simulink library "libreria_comunicaciones_cliente1T"  (R2018a)
settings: Solver=VariableStepAuto  StartTime=0.0  StopTime=10.0  RelTol=1e-3
undefined symbols (not defined in the file or in its folder): Ts
libraries: simulink x1
settings Model: Creator=ana-n  LastModifiedBy=ana-n
settings CodeAppCC: StateflowObjectComments=on

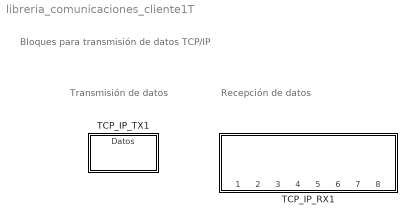
== system libreria_comunicaciones_cliente1T ==
  note: Bloques para transmisión de datos TCP/IP
  note: Recepción de datos
  note: Transmisión de datos
  TCP_IP_RX1 : Subsystem
      mask Display:
      | disp('TCP_IP_RX')
      | port_label('output',1,'RL1');
      | port_label('output',2,'RL2');
      | port_label('output',3,'RL3');
      | port_label('output',4,'RL4');
      | port_label('output',5,'RL5');
      | port_label('output',6,'Top');
      | port_label('output',7,'Top_graf');
      | port_label('output',8,'add');
  TCP_IP_TX1 : Subsystem
      mask Display: disp('TCP_IP_TX');

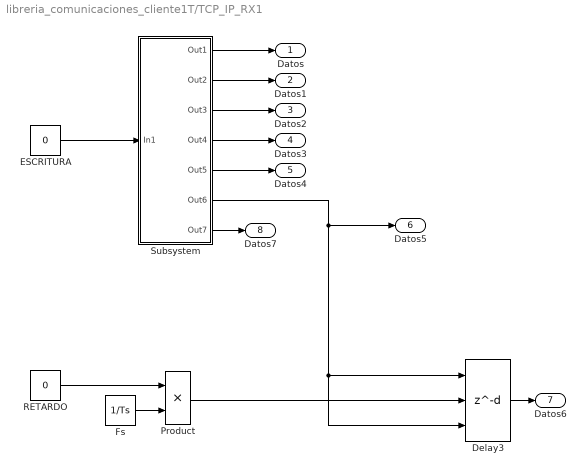
== system libreria_comunicaciones_cliente1T/TCP_IP_RX1 ==
  Delay3 : Delay  DelayLengthSource=Input port  DelayLength=1  DelayLengthUpperLimit=1000  InitialConditionSource=Input port  InitialCondition=0  InputProcessing=Inherited
      settings: InputPortMap=u0,p1,p4
  ESCRITURA : Constant  Value=0
  Fs : Constant  Value=1/Ts
  Product : Product
  RETARDO : Constant  Value=0
  Subsystem : Subsystem
      mask Display: disp('demux')
  Datos : Outport
  Datos1 : Outport  Port=2
  Datos2 : Outport  Port=3
  Datos3 : Outport  Port=4
  Datos4 : Outport  Port=5
  Datos5 : Outport  Port=6
  Datos6 : Outport  Port=7
  Datos7 : Outport  Port=8
  wires:
  Product/1 -> Delay3/2
  RETARDO/1 -> Product/1
  Fs/1 -> Product/2
  ESCRITURA/1 -> Subsystem/1(In1)
  Subsystem/1(Out1) -> Datos/1
  Subsystem/2(Out2) -> Datos1/1
  Subsystem/3(Out3) -> Datos2/1
  Subsystem/4(Out4) -> Datos3/1
  Subsystem/5(Out5) -> Datos4/1
  Subsystem/6(Out6) -> Datos5/1, Delay3/1, Delay3/3
  Delay3/1 -> Datos6/1
  Subsystem/7(Out7) -> Datos7/1

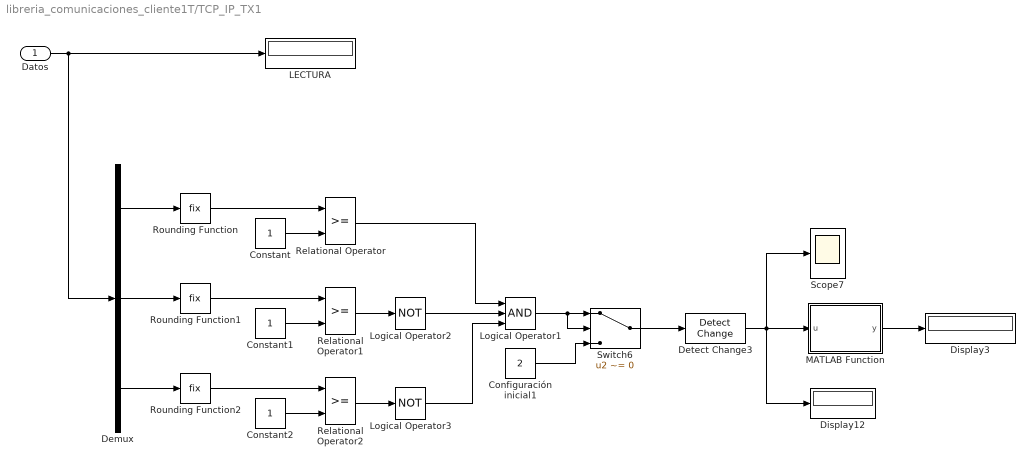
== system libreria_comunicaciones_cliente1T/TCP_IP_TX1 ==
  Datos : Inport
  Configuración inicial1 : Constant  Value=2
  Constant : Constant
  Constant1 : Constant
  Constant2 : Constant
  Demux : Demux  Outputs=3
  Detect Change3 : simulink/Logic and Bit Operations/Detect Change  vinit=0  OutDataTypeStr=boolean
  Display12 : Display
  Display3 : Display
  LECTURA : Display
  Logical Operator1 : Logic  Inputs=3  AllPortsSameDT=off  OutDataTypeStr=boolean
  Logical Operator2 : Logic  Operator=NOT  Inputs=3  AllPortsSameDT=off  OutDataTypeStr=boolean
  Logical Operator3 : Logic  Operator=NOT  Inputs=3  AllPortsSameDT=off  OutDataTypeStr=boolean
  MATLAB Function : MATLAB Function  TreatAsAtomicUnit=on
  Relational Operator : RelationalOperator  OutDataTypeStr=boolean  RndMeth=Simplest
  Relational Operator1 : RelationalOperator  OutDataTypeStr=boolean  RndMeth=Simplest
  Relational Operator2 : RelationalOperator  OutDataTypeStr=boolean  RndMeth=Simplest
  Rounding Function : Rounding  Operator=fix
  Rounding Function1 : Rounding  Operator=fix
  Rounding Function2 : Rounding  Operator=fix
  Scope7 : Scope
  Switch6 : Switch  Criteria=u2 ~= 0
  wires:
  MATLAB Function/1(y) -> Display3/1
  Datos/1 -> Demux/1, LECTURA/1
  Demux/1 -> Rounding Function/1
  Demux/2 -> Rounding Function1/1
  Demux/3 -> Rounding Function2/1
  Switch6/1 -> Detect Change3/1
  Detect Change3/1 -> MATLAB Function/1(u), Display12/1, Scope7/1
  Relational Operator1/1 -> Logical Operator2/1
  Constant1/1 -> Relational Operator1/2
  Rounding Function1/1 -> Relational Operator1/1
  Rounding Function2/1 -> Relational Operator2/1
  Constant/1 -> Relational Operator/2
  Constant2/1 -> Relational Operator2/2
  Logical Operator1/1 -> Switch6/2, Switch6/1
  Rounding Function/1 -> Relational Operator/1
  Configuración inicial1/1 -> Switch6/3
  Logical Operator2/1 -> Logical Operator1/2
  Logical Operator3/1 -> Logical Operator1/3
  Relational Operator/1 -> Logical Operator1/1
  Relational Operator2/1 -> Logical Operator3/1

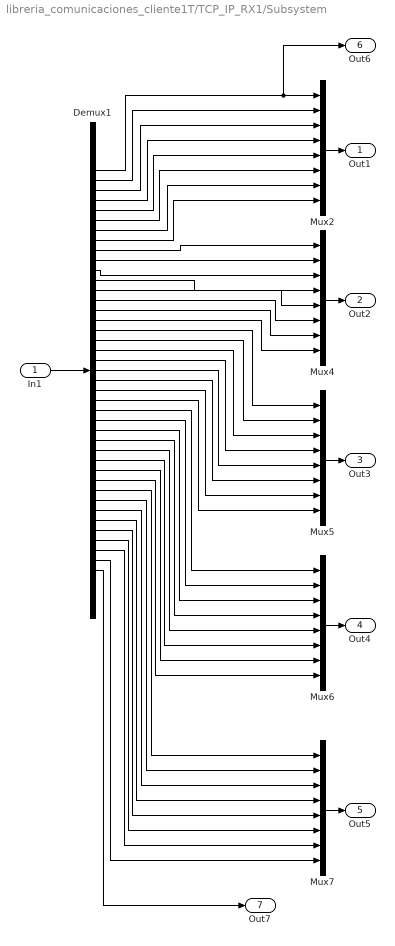
== system libreria_comunicaciones_cliente1T/TCP_IP_RX1/Subsystem ==
  In1 : Inport
  Demux1 : Demux  Outputs=41
  Mux{2,4..7} (5 alike) : Mux  Inputs=8
  Out1 : Outport
  Out2 : Outport  Port=2
  Out3 : Outport  Port=3
  Out4 : Outport  Port=4
  Out5 : Outport  Port=5
  Out6 : Outport  Port=6
  Out7 : Outport  Port=7
  wires:
  Demux1/33 -> Mux7/1
  Demux1/36 -> Mux7/4
  Demux1/6 -> Mux2/6
  Demux1/22 -> Mux5/6
  Demux1/30 -> Mux6/6
  Demux1/34 -> Mux7/2
  Demux1/16 -> Mux4/8
  Demux1/31 -> Mux6/7
  Mux4/1 -> Out2/1
  Mux5/1 -> Out3/1
  Mux2/1 -> Out1/1
  Demux1/14 -> Mux4/6
  Demux1/24 -> Mux5/8
  Demux1/39 -> Mux7/7
  Demux1/3 -> Mux2/3
  Demux1/40 -> Mux7/8
  Demux1/38 -> Mux7/6
  Demux1/12 -> Mux4/4
  Demux1/35 -> Mux7/3
  Demux1/18 -> Mux5/2
  Demux1/1 -> Out6/1, Mux2/1
  Demux1/5 -> Mux2/5
  Demux1/19 -> Mux5/3
  Demux1/37 -> Mux7/5
  Demux1/8 -> Mux2/8
  Demux1/29 -> Mux6/5
  Demux1/28 -> Mux6/4
  Demux1/11 -> Mux4/3
  Demux1/27 -> Mux6/3
  Demux1/26 -> Mux6/2
  Demux1/25 -> Mux6/1
  Demux1/15 -> Mux4/7
  Demux1/17 -> Mux5/1
  Demux1/10 -> Mux4/2
  Demux1/13 -> Mux4/5
  Demux1/9 -> Mux4/1
  Demux1/4 -> Mux2/4
  Demux1/21 -> Mux5/5
  Demux1/7 -> Mux2/7
  Demux1/2 -> Mux2/2
  Demux1/20 -> Mux5/4
  Demux1/32 -> Mux6/8
  Mux7/1 -> Out5/1
  Demux1/23 -> Mux5/7
  Mux6/1 -> Out4/1
  In1/1 -> Demux1/1
  Demux1/41 -> Out7/1

== matlab function libreria_comunicaciones_cliente1T/TCP_IP_TX1/MATLAB Function ==
  data: u input; y output
%Esta función envía y recibos los datos
%desde el CCL a través del script_ciclo_vs.m
function y = fcn(u)
    coder.extrinsic('run')
    if u==1
        run script_ciclo_vs1.m
        y=1;
    else
        y=0;
    end
end
